simulink model "motor"  (R2022a)
settings: Solver=VariableStepAuto  StartTime=0.0  StopTime=10.0  RelTol=1e-3
values from neighbouring files (symbols this model uses):
  beta = 12e-4    (= 0.0012)    [parametrosmotor.m]
  J = 1.07e-3    (= 0.00107)    [parametrosmotor.m]
  Kt = 0.0235    [parametrosmotor.m]
  Kv = 0.02352    [parametrosmotor.m]
  L = 0.0238    [parametrosmotor.m]
  R = 2.06    [parametrosmotor.m]
  Tl = 0.03    [parametrosmotor.m]
settings Model: Creator=fermo  LastModifiedBy=fermo

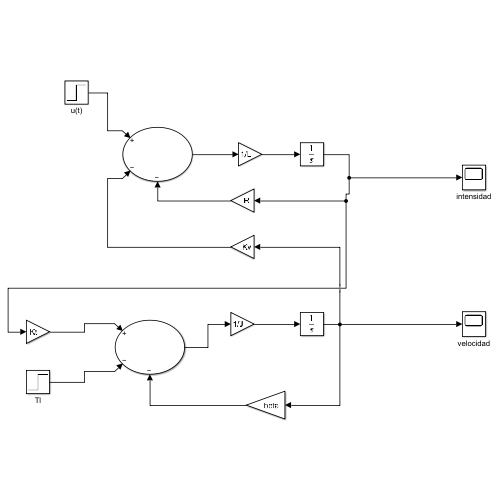
[thumbnail: Simulink's stored preview of the top-level diagram]
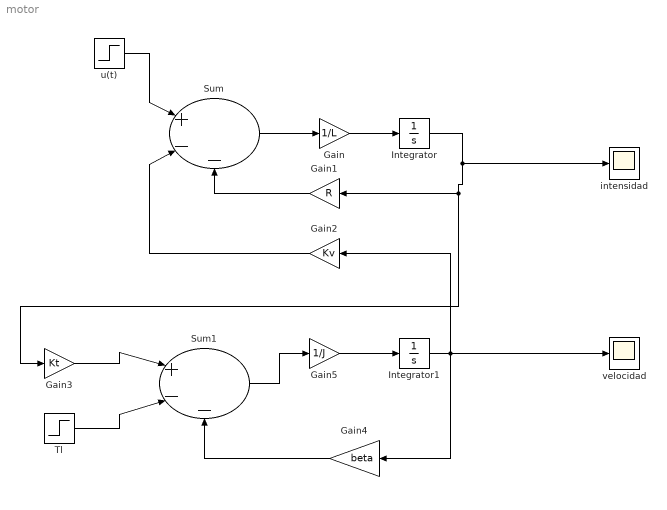
== system motor ==
  Gain : Gain  Gain=1/L
  Gain1 : Gain  Gain=R
  Gain2 : Gain  Gain=Kv
  Gain3 : Gain  Gain=Kt
  Gain4 : Gain  Gain=beta
  Gain5 : Gain  Gain=1/J
  Integrator : Integrator
  Integrator1 : Integrator
  Sum : Sum  Inputs=|+--
  Sum1 : Sum  Inputs=|+--
  Tl : Step  Time=6  After=Tl  SampleTime=0
  intensidad : Scope
  u(t) : Step  After=12  SampleTime=0
  velocidad : Scope
  wires:
  Sum/1 -> Gain/1
  Gain/1 -> Integrator/1
  Gain1/1 -> Sum/3
  Gain2/1 -> Sum/2
  Gain3/1 -> Sum1/1
  Gain4/1 -> Sum1/3
  Sum1/1 -> Gain5/1
  Gain5/1 -> Integrator1/1
  u(t)/1 -> Sum/1
  Integrator/1 -> intensidad/1, Gain3/1, Gain1/1
  Integrator1/1 -> velocidad/1, Gain4/1, Gain2/1
  Tl/1 -> Sum1/2
